simulink model "SelfBalancedRobot"  (R2018a)
settings: Solver=VariableStepAuto  StartTime=0.0  StopTime=15  RelTol=1e-3
undefined symbols (not defined in the file or in its folder): I, l, m, M
libraries: dspstat3 x1, simulink x1
settings Model: Creator=baixiao  LastModifiedBy=baixiao

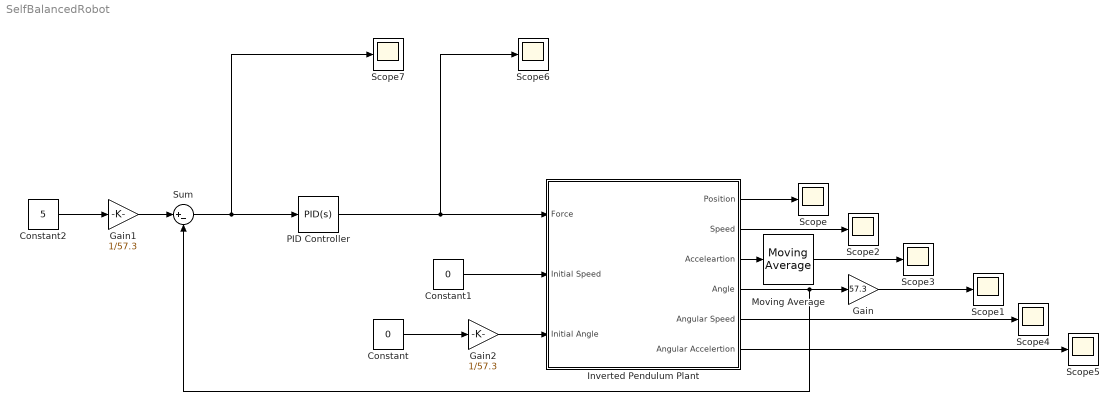
== system SelfBalancedRobot ==
  Constant : Constant  Value=0
  Constant1 : Constant  Value=0
  Constant2 : Constant  Value=5
  Gain : Gain  Gain=57.3
  Gain1 : Gain  Gain=1/57.3
  Gain2 : Gain  Gain=1/57.3
  Inverted Pendulum Plant : Subsystem
  Moving Average : dspstat3/Moving Average  Method=Sliding window  ForgettingFactorPort=off  SpecifyWindowLength=on  WindowLength=100  ForgettingFactor=0.9  SimulateUsing=Code generation
  PID Controller : simulink/Continuous/PID Controller  Controller=PID  TimeDomain=Continuous-time  SampleTime=-1  IntegratorMethod=Forward Euler  FilterMethod=Forward Euler  Form=Parallel  UseFilter=on  ControllerParametersSource=internal  P=547.943211410278  I=5.63040871500577  D=527  N=150.998712012709  InitialConditionSource=internal  InitialConditionForIntegrator=0  InitialConditionForFilter=0  ExternalReset=none  LimitOutput=on  UpperSaturationLimit=1  LowerSaturationLimit=-1  LinearizeAsGain=on  AntiWindupMode=none  Kb=1  TrackingMode=off  Kt=1  PParamMin=[]  PParamMax=[]  IParamMin=[]  IParamMax=[]  DParamMin=[]  DParamMax=[]  NParamMin=[]  NParamMax=[]  KbParamMin=[]  KbParamMax=[]  KtParamMin=[]  KtParamMax=[]  POutMin=[]  POutMax=[]  IOutMin=[]  IOutMax=[]  DOutMin=[]  DOutMax=[]  NOutMin=[]  NOutMax=[]  KbOutMin=[]  KbOutMax=[]  KtOutMin=[]  KtOutMax=[]  IntegratorOutMin=[]  IntegratorOutMax=[]  FilterOutMin=[]  FilterOutMax=[]  SumOutMin=[]  SumOutMax=[]  SumI1OutMin=[]  SumI1OutMax=[]  SumI2OutMin=[]  SumI2OutMax=[]  SumI3OutMin=[]  SumI3OutMax=[]  SumDOutMin=[]  SumDOutMax=[]  SaturationOutMin=[]  SaturationOutMax=[]  IntegratorContinuousStateAttributes=''  IntegratorStateMustResolveToSignalObject=off  IntegratorRTWStateStorageClass=Auto  FilterContinuousStateAttributes=''  FilterStateMustResolveToSignalObject=off  FilterRTWStateStorageClass=Auto  DifferentiatorICPrevScaledInput=0  DifferentiatorOutMin=[]  DifferentiatorOutMax=[]  FilterDiffOutCoefMin=[]  FilterDiffOutCoefMax=[]  SumDenOutMin=[]  SumDenOutMax=[]  SumNumOutMin=[]  SumNumOutMax=[]  ReciprocalOutMin=[]  ReciprocalOutMax=[]  DivideOutMin=[]  DivideOutMax=[]  TunerSelectOption=Transfer Function Based (PID Tuner App)
  Scope{,1..7} (8 alike) : Scope
  Sum : Sum  Inputs=|+-
  wires:
  Constant/1 -> Gain2/1
  Constant1/1 -> Inverted Pendulum Plant/2(Initial Speed)
  Inverted Pendulum Plant/1(Position) -> Scope/1
  Inverted Pendulum Plant/2(Speed) -> Scope2/1
  Inverted Pendulum Plant/3(Acceleartion) -> Moving Average/1
  Inverted Pendulum Plant/4(Angle) -> Sum/2, Gain/1
  Inverted Pendulum Plant/5(Angular Speed) -> Scope4/1
  Inverted Pendulum Plant/6(Angular Accelertion) -> Scope5/1
  Constant2/1 -> Gain1/1
  Gain/1 -> Scope1/1
  Gain1/1 -> Sum/1
  Sum/1 -> PID Controller/1, Scope7/1
  PID Controller/1 -> Inverted Pendulum Plant/1(Force), Scope6/1
  Gain2/1 -> Inverted Pendulum Plant/3(Initial Angle)
  Moving Average/1 -> Scope3/1

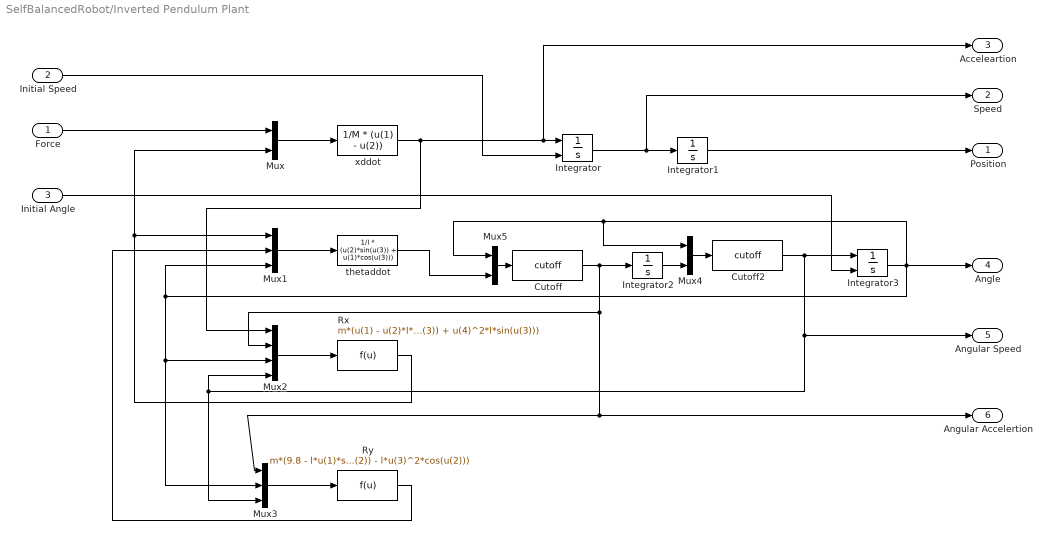
== system SelfBalancedRobot/Inverted Pendulum Plant ==
  Force : Inport
  Initial Speed : Inport  Port=2
  Initial Angle : Inport  Port=3
  Cutoff : MATLABFcn  MATLABFcn=cutoff
  Cutoff2 : MATLABFcn  MATLABFcn=cutoff
  Integrator : Integrator  InitialConditionSource=external
  Integrator1 : Integrator
  Integrator2 : Integrator
  Integrator3 : Integrator  InitialConditionSource=external  InitialCondition=0.1
  Mux : Mux  Inputs=2
  Mux1 : Mux  Inputs=3
  Mux2 : Mux
  Mux3 : Mux  Inputs=3
  Mux4 : Mux  Inputs=2
  Mux5 : Mux  Inputs=2
  Rx : Fcn  Expr=m*(u(1) - u(2)*l*cos(u(3)) + u(4)^2*l*sin(u(3)))
  Ry : Fcn  Expr=m*(9.8 - l*u(1)*sin(u(2)) - l*u(3)^2*cos(u(2)))
  thetaddot : Fcn  Expr=1/I * (u(2)*sin(u(3)) + u(1)*cos(u(3)))
  xddot : Fcn  Expr=1/M * (u(1) - u(2))
  Position : Outport
  Speed : Outport  Port=2
  Acceleartion : Outport  Port=3
  Angle : Outport  Port=4
  Angular Speed : Outport  Port=5
  Angular Accelertion : Outport  Port=6
  wires:
  Mux2/1 -> Rx/1
  Integrator1/1 -> Position/1
  Mux4/1 -> Cutoff2/1
  Mux5/1 -> Cutoff/1
  Force/1 -> Mux/1
  Integrator/1 -> Speed/1, Integrator1/1
  Initial Speed/1 -> Integrator/2
  Mux3/1 -> Ry/1
  xddot/1 -> Acceleartion/1, Integrator/1, Mux2/1
  Cutoff2/1 -> Angular Speed/1, Mux3/3, Mux2/4, Integrator3/1
  Mux1/1 -> thetaddot/1
  Initial Angle/1 -> Integrator3/2
  thetaddot/1 -> Mux5/2
  Cutoff/1 -> Angular Accelertion/1, Mux3/1, Mux2/2, Integrator2/1
  Mux/1 -> xddot/1
  Ry/1 -> Mux1/2
  Integrator3/1 -> Angle/1, Mux1/3, Mux2/3, Mux3/2, Mux4/1, Mux5/1
  Rx/1 -> Mux1/1, Mux/2
  Integrator2/1 -> Mux4/2
